simulink model "MagLevS"  (R2020b)
settings: Solver=ode4  StartTime=0.0  StopTime=0.5  FixedStep=0.000001  RelTol=1e-3
settings Model: Creator=Aravindsamy  LastModifiedBy=Aravindsamy

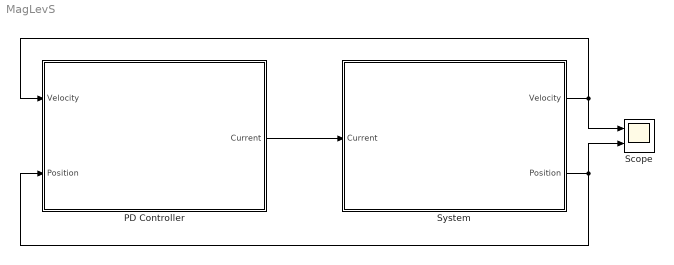
== system MagLevS ==
  PD Controller : Subsystem  mask{Xref=-0.009, Kd=4, Kp=300}
      mask prompts: Xref "Position Reference"; Kd "Differential Gain"; Kp "Proportional Gain"
      mask Display: disp('i=Kp(xref-x)+Kd(-vx)', 'texmode', 'on')
  Scope : Scope  NumInputPorts=2
  System : Subsystem  mask{ipm=2, x=0.009, m=0.06, g=9.81, Kf=1.192e-5, x0=-0.009, v0=0}
      mask prompts: ipm "Permanent Magnet Current"; x "Position"; m "Mass"; g "Gravity"; x0 "Initial Position"; v0 "InitialVelocity"
      mask Display: disp('Fmg=((Kf/m)*sq((i+ipm)/x))', 'texmode', 'on')
  wires:
  PD Controller/1(Current) -> System/1(Current)
  System/2(Position) -> Scope/2, PD Controller/2(Position)
  System/1(Velocity) -> Scope/1, PD Controller/1(Velocity)

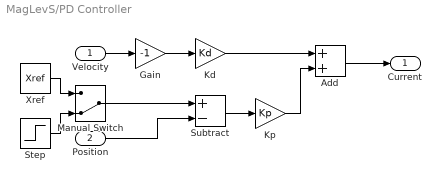
== system MagLevS/PD Controller ==
  Velocity : Inport
  Position : Inport  Port=2
  Add : Sum
  Gain : Gain  Gain=-1
  Kd : Gain  Gain=Kd
  Kp : Gain  Gain=Kp
  Manual Switch : ManualSwitch  CurrentSetting=0
  Step : Step  Time=0.1  Before=-0.009  After=-0.0095  SampleTime=0
  Subtract : Sum  Inputs=+-
  Xref : Constant  Value=Xref
  Current : Outport
  wires:
  Velocity/1 -> Gain/1
  Gain/1 -> Kd/1
  Position/1 -> Subtract/2
  Subtract/1 -> Kp/1
  Kd/1 -> Add/1
  Kp/1 -> Add/2
  Add/1 -> Current/1
  Step/1 -> Manual Switch/2
  Manual Switch/1 -> Subtract/1
  Xref/1 -> Manual Switch/1

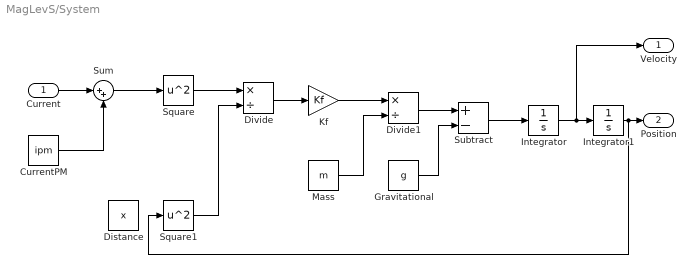
== system MagLevS/System ==
  Current : Inport
  CurrentPM : Constant  Value=ipm
  Distance : Constant  Value=x
  Divide : Product  Inputs=*/
  Divide1 : Product  Inputs=*/
  Gravitational : Constant  Value=g
  Integrator : Integrator  InitialCondition=v0
  Integrator1 : Integrator  InitialCondition=x0
  Kf : Gain  Gain=Kf
  Mass : Constant  Value=m
  Square : Math  Operator=square  SaturateOnIntegerOverflow=on
  Square1 : Math  Operator=square  SaturateOnIntegerOverflow=on
  Subtract : Sum  Inputs=+-
  Sum : Sum  Inputs=|++
  Velocity : Outport
  Position : Outport  Port=2
  wires:
  Current/1 -> Sum/1
  CurrentPM/1 -> Sum/2
  Sum/1 -> Square/1
  Square/1 -> Divide/1
  Square1/1 -> Divide/2
  Divide/1 -> Kf/1
  Kf/1 -> Divide1/1
  Mass/1 -> Divide1/2
  Subtract/1 -> Integrator/1
  Integrator/1 -> Integrator1/1, Velocity/1
  Integrator1/1 -> Square1/1, Position/1
  Divide1/1 -> Subtract/1
  Gravitational/1 -> Subtract/2
